simulink model "traffic_light_sim"  (R2024b)
settings: Solver=FixedStepAuto  StartTime=0.0  StopTime=100  FixedStep=0.1  RelTol=1e-3
settings Model: Creator=nelsenyoung  LastModifiedBy=nelsenyoung

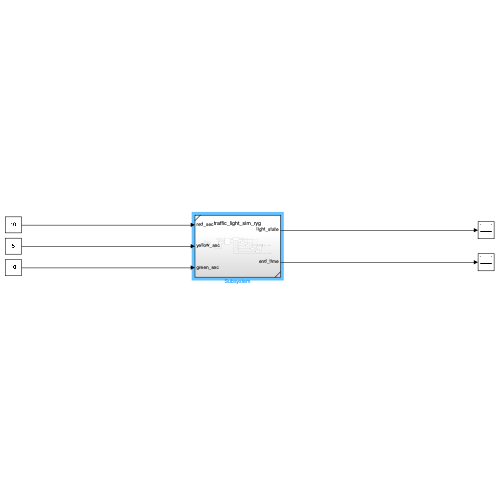
[thumbnail: Simulink's stored preview of the top-level diagram]
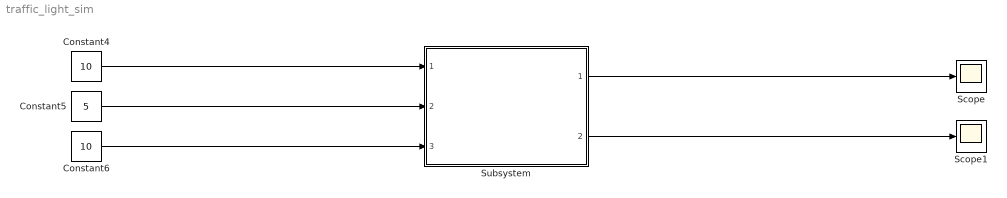
== system traffic_light_sim ==
  Constant4 : Constant  Value=10
  Constant5 : Constant  Value=5
  Constant6 : Constant  Value=10
  Scope : Scope
  Scope1 : Scope
  Subsystem : Subsystem  ReferencedSubsystem=traffic_light_sim_ryg
  wires:
  Constant4/1 -> Subsystem/1
  Constant5/1 -> Subsystem/2
  Constant6/1 -> Subsystem/3
  Subsystem/1 -> Scope/1
  Subsystem/2 -> Scope1/1
